simulink model "Baseline_Ctrl"  (R2020a)
settings: Solver=FixedStepAuto  StartTime=0.0  StopTime=10.0  FixedStep=DT  RelTol=1e-3
values from neighbouring files (symbols this model uses):
  K_T = 0.5e-6*pi*tp.rho*tp.R^5*tp.C_p_star/(tp.lambda_star^3)    [baseline_design.m]    (also in run_Top_Model.m)
  tp = turbine_params_5MW()    [baseline_design.m]    (also in run_Top_Model.m)
settings Model: Creator=lpwoolcock  LastModifiedBy=lpwoolcock

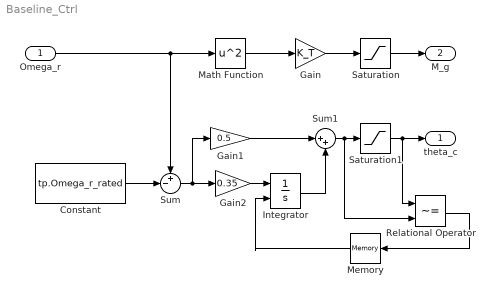
== system Baseline_Ctrl ==
  Omega_r : Inport
  Constant : Constant  Value=tp.Omega_r_rated
  Gain : Gain  Gain=K_T
  Gain1 : Gain  Gain=0.5
  Gain2 : Gain  Gain=0.35
  Integrator : Integrator  ExternalReset=level  LowerSaturationLimit=0
  Math Function : Math  Operator=square  SaturateOnIntegerOverflow=on
  Memory : Memory
  Relational Operator : RelationalOperator  Operator=~=  OutDataTypeStr=boolean  RndMeth=Simplest
  Saturation : Saturate  UpperLimit=tp.M_g_rated  LowerLimit=-tp.M_g_rated
  Saturation1 : Saturate  UpperLimit=inf  LowerLimit=0
  Sum : Sum  Inputs=+-|
  Sum1 : Sum  Inputs=|++
  theta_c : Outport
  M_g : Outport  Port=2
  wires:
  Math Function/1 -> Gain/1
  Omega_r/1 -> Sum/1, Math Function/1
  Gain/1 -> Saturation/1
  Saturation1/1 -> Relational Operator/1, theta_c/1
  Saturation/1 -> M_g/1
  Constant/1 -> Sum/2
  Sum/1 -> Gain1/1, Gain2/1
  Gain2/1 -> Integrator/1
  Gain1/1 -> Sum1/1
  Integrator/1 -> Sum1/2
  Sum1/1 -> Relational Operator/2, Saturation1/1
  Relational Operator/1 -> Memory/1
  Memory/1 -> Integrator/2
